simulink model "Model_aaron"  (R2026a)
settings: Solver=VariableStepAuto  StopTime=10  RelTol=1e-2  AbsTol=1e-2  EnableMultiTasking=on
values from neighbouring files (symbols this model uses):
  N = zeros(6,3)    [script_aaron.m]    (also in sea_sim.m = 100)
  s = 10    [sea_sim.m]
  Tinv = pinv(T)    [script_aaron.m]
  Ts = 0.01    [script_aaron.m]
undefined symbols (not defined in the file or in its folder): Kd_heave, Kd_pitch, Kd_roll, Ki_heave, Ki_pitch, Ki_roll, Kp_heave, Kp_pitch, Kp_roll, X, Y, Z
libraries: sm_lib x75, nesl_utility x14, slpidlib x3, simulink x3
(part 4 of 4)

== matlab function Model_aaron/PLANTA/INVERSE  KINEMATICS ==
  settings: updateMethod=DISCRETE
  data: dL output; alpha input; theta input; z input; L output; L0 output; R_TOP input
function [dL, L, L0] = marlup_ik(alpha, theta, z, R_TOP)
%MARLUP_IK  Cinematica inversa de MARLUP: (roll, pitch, heave) -> pistones.
%
%   [dL, L, L0] = MARLUP_IK(alpha, theta, z)
%
%   El calculo depende UNICAMENTE de la geometria de los anclajes:
%   radio inferior, radio superior y altura nominal entre soportes.
%   Ninguna caracteristica del piston (carrera, longitud, modelo) interviene.
%
%   ENTRADAS
%     alpha : roll  [rad]  giro alrededor de x
%     theta : pitch [rad]  giro alrededor de y
%     z     : [m]  separacion vertical COMANDADA entre el plano de anclaje
%                  del SORPOTE (abajo) y el del TRIANGULO (arriba).
%                  En la pose ensamblada vale Z0.
%
%   SALIDAS
%     dL : 3x1 [m]  ESTA es la que va a los Prismatic Joint. Desplazamiento
%                   respecto de la pose ensamblada del CAD. Vale [0;0;0]
%                   exactamente cuando alpha=theta=0 y z=Z0.
%     L  : 3x1 [m]  distancia entre centros de rotula (diagnostico).
%     L0 : 1x1 [m]  distancia nominal, DERIVADA de la geometria.
%
%   ORDEN: indice 1 <-> F1 (phi=-30), 2 <-> F2 (phi=90), 3 <-> F3 (phi=210),
%   el mismo de las columnas de T en Script_MARLUP_Final.m.
%
%   Modelo:  T_0^P = Trasl(0,0,z) * Ry(theta) * Rx(alpha)
%            L_i   = || T_0^P * p_i^P  -  b_i ||
%#codegen

% ============ UNICOS PARAMETROS: medirlos en el ensamblaje CAD ===========
R_BASE = 0.7608;   % [m] radio del anclaje inferior (SORPOTE), eje -> centro rotula
%R_TOP  = 0.143;   % [m] radio del anclaje superior (TRIANGULO), idem
Z0     = 1.377;   % [m] separacion vertical entre ambos planos, pose ensamblada
% =========================================================================

PHI = [-30; 90; 210] * pi/180;      % distribucion angular de los tres brazos

DR = R_BASE - R_TOP;
L0 = sqrt(DR*DR + Z0*Z0);           % longitud nominal: RESULTADO, no dato

ca = cos(alpha);  sa = sin(alpha);
ct = cos(theta);  st = sin(theta);

R = [  ct,  sa*st,  ca*st ;         % Ry(theta)*Rx(alpha)
        0,     ca,    -sa ;
      -st,  sa*ct,  ca*ct ];

L = zeros(3,1);
for i = 1:3
    cp = cos(PHI(i));
    sp = sin(PHI(i));

    b  = [R_BASE*cp; R_BASE*sp; 0];   % anclaje inferior, fijo en la base
    pP = [R_TOP*cp;  R_TOP*sp;  0];   % anclaje superior, en el marco movil
    d  = R*pP + [0; 0; z] - b;

    L(i) = sqrt(d(1)*d(1) + d(2)*d(2) + d(3)*d(3));
end

dL = L - L0;
end
